simulink model "Yaw_Control_Diff_TS9"  (Simulink 7.6)
settings: Solver=ode45  SolverMode=SingleTasking  StartTime=0  StopTime=10  FixedStep=0.002  RelTol=1e-3  AbsTol=1e-6
libraries: Solver_SF x1
settings Model: Creator=pmather  LastModifiedBy=mkhan  ExtModeTrigMode=oneshot  ExtModeArmWhenConnect=off
settings DataIOCC: LimitDataPoints=off  SignalLoggingName=sigsOut
settings OptimizationCC: BlockReduction=off  BooleanDataType=off
settings DebuggingCC: SaveWithParameterizedLinksMsg=none  SignalResolutionControl=TryResolveAllWithWarning  SolverPrmCheckMsg=none  MultiTaskDSMMsg=warning  MultiTaskCondExecSysMsg=none  StrictBusMsg=None
settings HardwareCC: TargetUnknown=on
settings RTWCC: TemplateMakefile=grt_vc.tmf  IncludeERTFirstTime=on

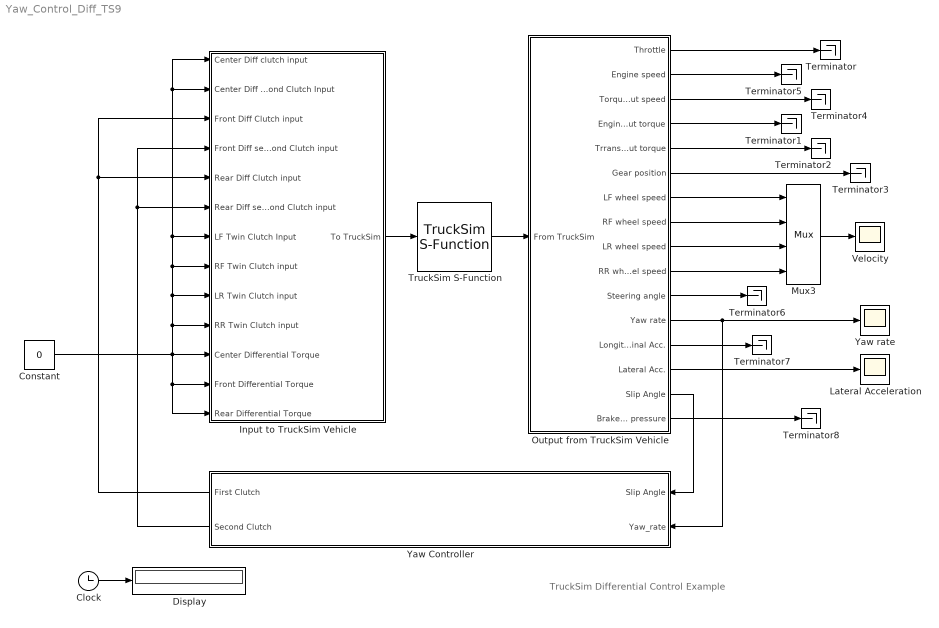
== system Yaw_Control_Diff_TS9 ==
  note: TruckSim Differential Control Example
  Clock : Clock
      settings: Decimation=10
  Constant : Constant  Value=0
  Display : Display
      settings: Format=bank  Decimation=100
  Input to TruckSim Vehicle : Subsystem
  Lateral Acceleration : Scope
      settings: TickLabels=on  YMin=-0.5  YMax=0.5  DataFormat=Array  SampleTime=100
  Mux3 : Mux
  Output from TruckSim Vehicle : Subsystem
  Terminator{,1..8} (9 alike) : Terminator
  TruckSim S-Function : Solver_SF/TruckSim S-Function  Priority=1  SIMFILE=simfile.sim
  Velocity : Scope
      settings: TickLabels=on  YMin=0  YMax=120  DataFormat=Array  SampleTime=100
  Yaw Controller : Subsystem  mask{YAW=0.24, CONTROL=1.2}
      mask prompts: YAW "Yaw Control Gain (-)"; CONTROL "Control Gain (-)"
  Yaw rate : Scope
      settings: TickLabels=on  YMin=-15  YMax=20  DataFormat=Array  SampleTime=100
  wires:
  Constant/1 -> Input to TruckSim Vehicle/11(Center Differential Torque), Input to TruckSim Vehicle/12("Front Differential Torque "), Input to TruckSim Vehicle/13(Rear Differential Torque), Input to TruckSim Vehicle/8(RF Twin Clutch input), Input to TruckSim Vehicle/7(LF Twin Clutch Input), Input to TruckSim Vehicle/2(Center Diff second Clutch Input), Input to TruckSim Vehicle/1(Center Diff clutch input), Input to TruckSim Vehicle/9(LR Twin Clutch input), Input to TruckSim Vehicle/10(RR Twin Clutch input)
  TruckSim S-Function/1 -> Output from TruckSim Vehicle/1(From TruckSim)
  Input to TruckSim Vehicle/1(To TruckSim) -> TruckSim S-Function/1
  Yaw Controller/1(First Clutch) -> Input to TruckSim Vehicle/3(Front Diff Clutch input), Input to TruckSim Vehicle/5(Rear Diff Clutch input)
  Yaw Controller/2(Second Clutch) -> Input to TruckSim Vehicle/4(Front Diff second Clutch input), Input to TruckSim Vehicle/6(Rear Diff second Clutch input)
  Clock/1 -> Display/1
  Mux3/1 -> Velocity/1
  Output from TruckSim Vehicle/7(LF wheel speed) -> Mux3/1
  Output from TruckSim Vehicle/8(RF wheel speed) -> Mux3/2
  Output from TruckSim Vehicle/9(LR wheel speed) -> Mux3/3
  Output from TruckSim Vehicle/10(RR wheel speed) -> Mux3/4
  Output from TruckSim Vehicle/1(Throttle) -> Terminator/1
  Output from TruckSim Vehicle/4(Engine output torque) -> Terminator1/1
  Output from TruckSim Vehicle/5(Trransmission output torque) -> Terminator2/1
  Output from TruckSim Vehicle/6(Gear position) -> Terminator3/1
  Output from TruckSim Vehicle/3(Torque converter output speed) -> Terminator4/1
  Output from TruckSim Vehicle/2(Engine speed) -> Terminator5/1
  Output from TruckSim Vehicle/11(Steering angle) -> Terminator6/1
  Output from TruckSim Vehicle/13(Longitudinal Acc.) -> Terminator7/1
  Output from TruckSim Vehicle/12(Yaw rate) -> Yaw rate/1, Yaw Controller/2(Yaw_rate)
  Output from TruckSim Vehicle/16(Brake M/C pressure) -> Terminator8/1
  Output from TruckSim Vehicle/14(Lateral Acc.) -> Lateral Acceleration/1
  Output from TruckSim Vehicle/15(Slip Angle) -> Yaw Controller/1(Slip Angle)

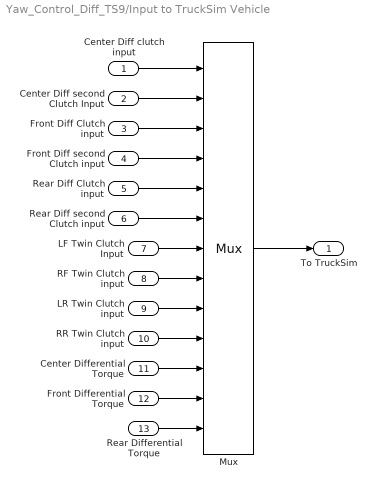
== system Yaw_Control_Diff_TS9/Input to TruckSim Vehicle ==
  Center Diff clutch input : Inport
  Center Diff second Clutch Input : Inport  Port=2
  Front Diff Clutch input : Inport  Port=3
  Front Diff second Clutch input : Inport  Port=4
  Rear Diff Clutch input : Inport  Port=5
  Rear Diff second Clutch input : Inport  Port=6
  LF Twin Clutch Input : Inport  Port=7
  RF Twin Clutch input : Inport  Port=8
  LR Twin Clutch input : Inport  Port=9
  RR Twin Clutch input : Inport  Port=10
  Center Differential Torque : Inport  Port=11
  "Front Differential Torque " : Inport  Port=12
  Rear Differential Torque : Inport  Port=13
  Mux : Mux  Inputs=13
  To TruckSim : Outport
  wires:
  Mux/1 -> To TruckSim/1
  Center Differential Torque/1 -> Mux/11
  Rear Differential Torque/1 -> Mux/13
  "Front Differential Torque "/1 -> Mux/12
  RR Twin Clutch input/1 -> Mux/10
  LR Twin Clutch input/1 -> Mux/9
  RF Twin Clutch input/1 -> Mux/8
  LF Twin Clutch Input/1 -> Mux/7
  Rear Diff second Clutch input/1 -> Mux/6
  Rear Diff Clutch input/1 -> Mux/5
  Front Diff second Clutch input/1 -> Mux/4
  Front Diff Clutch input/1 -> Mux/3
  Center Diff second Clutch Input/1 -> Mux/2
  Center Diff clutch input/1 -> Mux/1

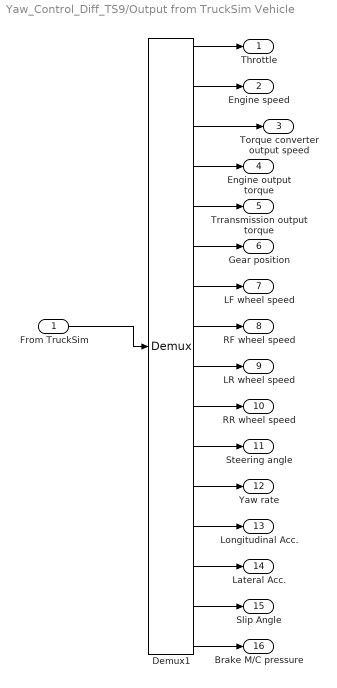
== system Yaw_Control_Diff_TS9/Output from TruckSim Vehicle ==
  From TruckSim : Inport
  Demux1 : Demux  Outputs=16
  Throttle : Outport
  Engine speed : Outport  Port=2
  Torque converter output speed : Outport  Port=3
  Engine output torque : Outport  Port=4
  Trransmission output torque : Outport  Port=5
  Gear position : Outport  Port=6
  LF wheel speed : Outport  Port=7
  RF wheel speed : Outport  Port=8
  LR wheel speed : Outport  Port=9
  RR wheel speed : Outport  Port=10
  Steering angle : Outport  Port=11
  Yaw rate : Outport  Port=12
  Longitudinal Acc. : Outport  Port=13
  Lateral Acc. : Outport  Port=14
  Slip Angle : Outport  Port=15
  Brake M/C pressure : Outport  Port=16
  wires:
  From TruckSim/1 -> Demux1/1
  Demux1/1 -> Throttle/1
  Demux1/2 -> Engine speed/1
  Demux1/3 -> Torque converter output speed/1
  Demux1/7 -> LF wheel speed/1
  Demux1/13 -> Longitudinal Acc./1
  Demux1/14 -> Lateral Acc./1
  Demux1/8 -> RF wheel speed/1
  Demux1/9 -> LR wheel speed/1
  Demux1/10 -> RR wheel speed/1
  Demux1/11 -> Steering angle/1
  Demux1/12 -> Yaw rate/1
  Demux1/4 -> Engine output torque/1
  Demux1/5 -> Trransmission output torque/1
  Demux1/6 -> Gear position/1
  Demux1/15 -> Slip Angle/1
  Demux1/16 -> Brake M/C pressure/1

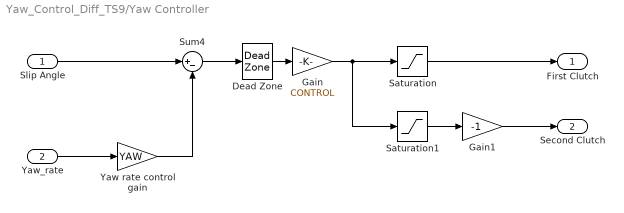
== system Yaw_Control_Diff_TS9/Yaw Controller ==
  Slip Angle : Inport
  Yaw_rate : Inport  Port=2
  Dead Zone : DeadZone  SaturateOnIntegerOverflow=on
  Gain : Gain  Gain=CONTROL  SaturateOnIntegerOverflow=on  OutDataTypeStr=Inherit: Same as input  ParamDataTypeStr=Inherit: Same as input
  Gain1 : Gain  Gain=-1  SaturateOnIntegerOverflow=on  OutDataTypeStr=Inherit: Same as input  ParamDataTypeStr=Inherit: Same as input
  Saturation : Saturate  UpperLimit=1  LowerLimit=0
  Saturation1 : Saturate  UpperLimit=0  LowerLimit=-1
  Sum4 : Sum  Inputs=|+-  SaturateOnIntegerOverflow=on  InputSameDT=on  OutDataTypeStr=Inherit: Same as first input
  Yaw rate control gain : Gain  Gain=YAW  SaturateOnIntegerOverflow=on  OutDataTypeStr=Inherit: Same as input  ParamDataTypeStr=Inherit: Same as input
  First Clutch : Outport
  Second Clutch : Outport  Port=2
  wires:
  Yaw rate control gain/1 -> Sum4/2
  Yaw_rate/1 -> Yaw rate control gain/1
  Dead Zone/1 -> Gain/1
  Sum4/1 -> Dead Zone/1
  Gain/1 -> Saturation/1, Saturation1/1
  Saturation1/1 -> Gain1/1
  Saturation/1 -> First Clutch/1
  Gain1/1 -> Second Clutch/1
  Slip Angle/1 -> Sum4/1
